simulink model "Centralized_Controller"  (R2023a)
settings: Solver=VariableStepAuto  StartTime=0.0  StopTime=10.0  RelTol=1e-3
libraries: simulink x1, dspinverses x1, DaVinci_LibDynamical x1
settings Model: Creator=afons  LastModifiedBy=afons

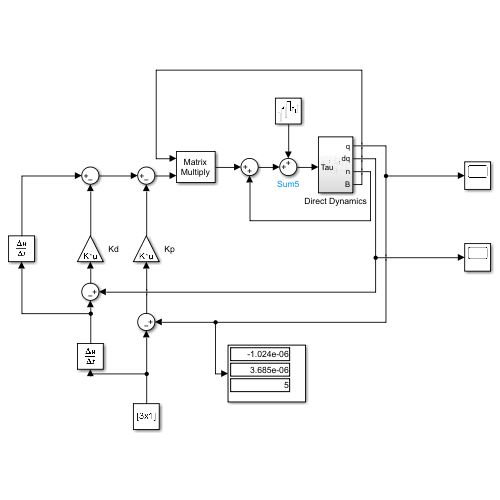
[thumbnail: Simulink's stored preview of the top-level diagram]
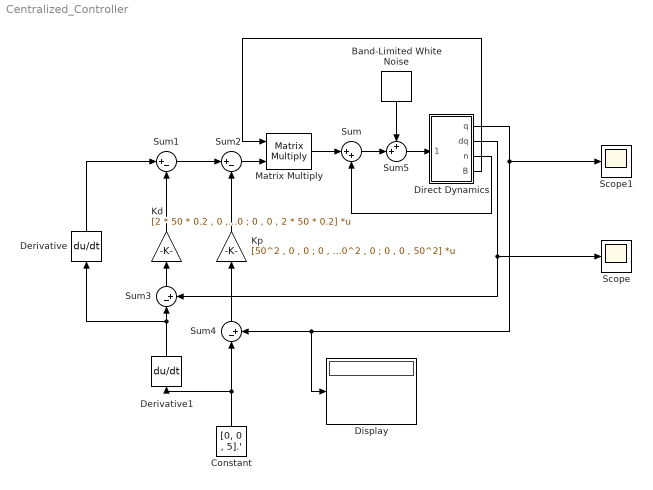
== system Centralized_Controller ==
  Band-Limited White Noise : simulink/Sources/Band-Limited White Noise  Cov=[0.1]  Ts=0.1  seed=[23341]
  Constant : Constant  Value=[0, 0 , 5].'
  Derivative : Derivative
  Derivative1 : Derivative
  Direct Dynamics : Subsystem
  Display : Display
  Kd : Gain  Gain=[2 * 50 * 0.2 , 0 , 0 ; 0 , 2 * 50 * 0.2 , 0 ; 0 , 0 , 2 * 50 * 0.2]  Multiplication=Matrix(K*u)
  Kp : Gain  Gain=[50^2 , 0 , 0 ; 0 , 50^2 , 0 ; 0 , 0 , 50^2]  Multiplication=Matrix(K*u)
  Matrix Multiply : Product  Multiplication=Matrix(*)
  Scope : Scope
  Scope1 : Scope
  Sum : Sum  Inputs=|++
  Sum1 : Sum  Inputs=|+-
  Sum2 : Sum  Inputs=|+-
  Sum3 : Sum  Inputs=|-+
  Sum4 : Sum  Inputs=|-+
  Sum5 : Sum  Inputs=++|
  wires:
  Matrix Multiply/1 -> Sum/1
  Sum2/1 -> Matrix Multiply/2
  Kp/1 -> Sum2/2
  Sum1/1 -> Sum2/1
  Kd/1 -> Sum1/2
  Sum3/1 -> Kd/1
  Sum4/1 -> Kp/1
  Direct Dynamics/1(q) -> Scope1/1, Display/1, Sum4/2
  Direct Dynamics/2(dq) -> Scope/1, Sum3/2
  Direct Dynamics/3(n) -> Sum/2
  Derivative1/1 -> Derivative/1, Sum3/1
  Constant/1 -> Derivative1/1, Sum4/1
  Derivative/1 -> Sum1/1
  Sum/1 -> Sum5/2
  Sum5/1 -> Direct Dynamics/1(Tau)
  Band-Limited White Noise/1 -> Sum5/1
  Direct Dynamics/4(B) -> Matrix Multiply/1

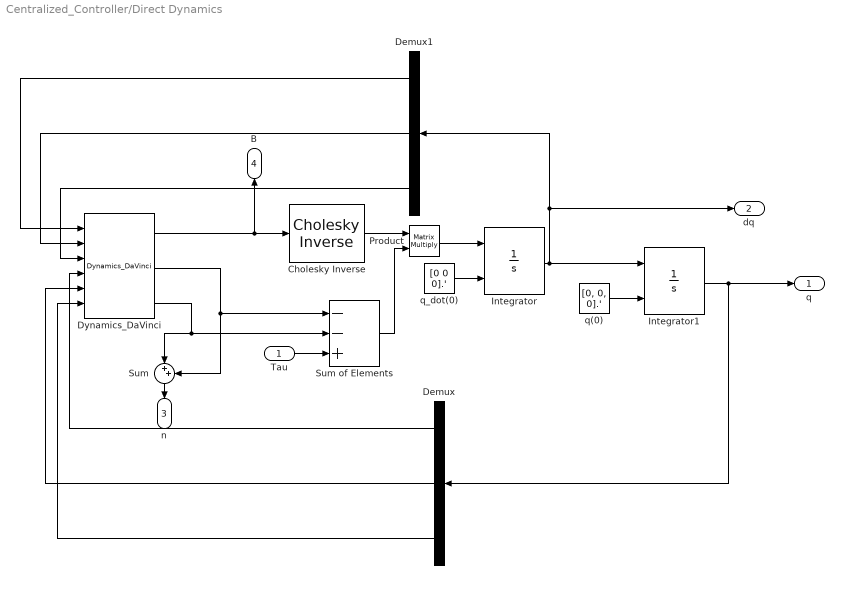
== system Centralized_Controller/Direct Dynamics ==
  Tau : Inport
  Cholesky Inverse : dspinverses/Cholesky Inverse  errmode=Warning
  Demux : Demux  Outputs=3
  Demux1 : Demux  Outputs=3
  Dynamics_DaVinci : DaVinci_LibDynamical/Dynamics_DaVinci  SystemSampleTime=-1  VariantActivationTime=update diagram  Latency=0  AutoFrameSizeCalculation=off
      settings: LibrarySourceBlock=|
      | simulink/User-Defined
      | Functions/MATLAB Function
  Integrator : Integrator  InitialConditionSource=external
  Integrator1 : Integrator  InitialConditionSource=external
  Product : Product  Multiplication=Matrix(*)
  Sum : Sum  Inputs=|++
  Sum of Elements : Sum  Inputs=--+
  q(0) : Constant  Value=[0, 0, 0].'
  q_dot(0) : Constant  Value=[0 0 0].'
  q : Outport
  dq : Outport  Port=2
  n : Outport  Port=3
  B : Outport  Port=4
  wires:
  Dynamics_DaVinci/2 -> Sum/2, Sum of Elements/1
  Integrator/1 -> dq/1, Demux1/1, Integrator1/1
  Product/1 -> Integrator/1
  Dynamics_DaVinci/3 -> Sum/1, Sum of Elements/2
  Integrator1/1 -> q/1, Demux/1
  Demux1/2 -> Dynamics_DaVinci/2
  Dynamics_DaVinci/1 -> B/1, Cholesky Inverse/1
  q_dot(0)/1 -> Integrator/2
  Sum of Elements/1 -> Product/2
  q(0)/1 -> Integrator1/2
  Demux/2 -> Dynamics_DaVinci/5
  Demux/3 -> Dynamics_DaVinci/6
  Demux/1 -> Dynamics_DaVinci/4
  Demux1/1 -> Dynamics_DaVinci/1
  Tau/1 -> Sum of Elements/3
  Demux1/3 -> Dynamics_DaVinci/3
  Cholesky Inverse/1 -> Product/1
  Sum/1 -> n/1
